simulink model "motor_control_SVPWM"  (R2023a)
settings: Solver=FixedStepAuto  StartTime=0.0  StopTime=10  FixedStep=1e-5  RelTol=1e-3
undefined symbols (not defined in the file): DiscIntNeverNeededParam
libraries: spsIGBTDiodeLib x6, simulink x3, spsCurrentMeasurementLib x3, spsAsynchronousMachineSIUnitsLib x1, spsDCVoltageSourceLib x1, slpidlib x1, spsTriangleGeneratorLib x1, sps_lib x1
settings Model: Creator=Vuong Thanh Tung  LastModifiedBy=Vuong Thanh Tung

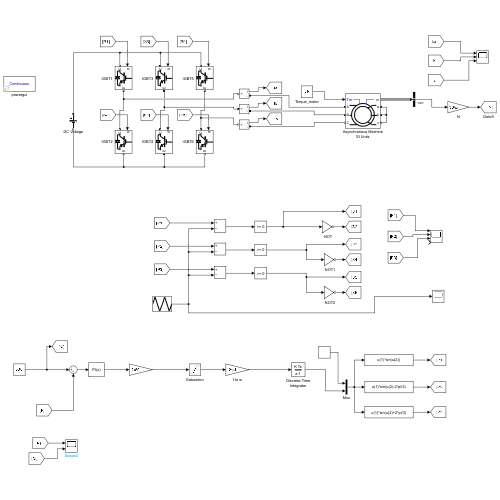
[thumbnail: Simulink's stored preview of the top-level diagram]
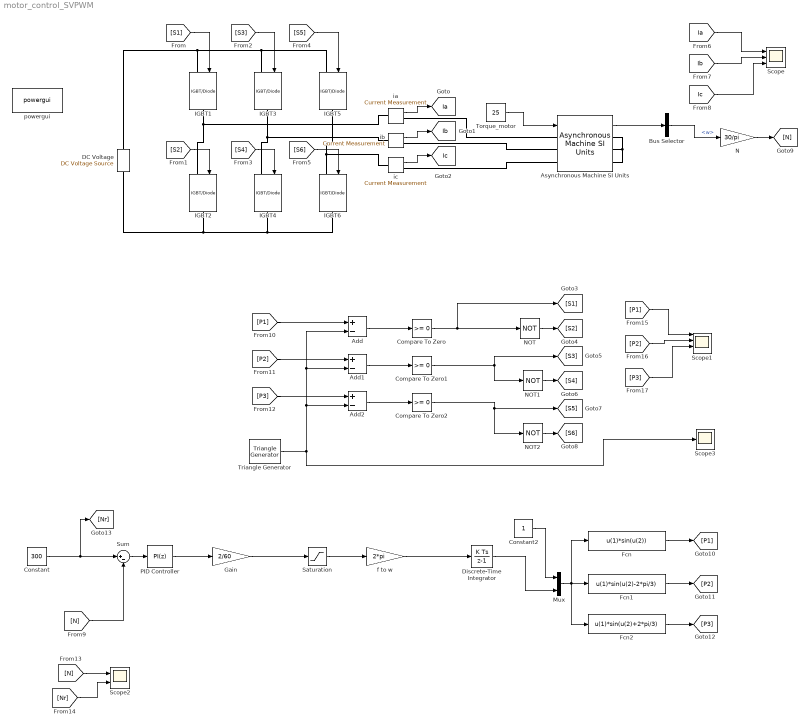
== system motor_control_SVPWM ==
  Add : Sum  Inputs=+-
  Add1 : Sum  Inputs=+-
  Add2 : Sum  Inputs=+-
  Asynchronous Machine SI Units : spsAsynchronousMachineSIUnitsLib/Asynchronous Machine SI Units  RotorType=Wound  PresetModel=No  MechanicalLoad=Torque Tm  ShowDetailedParameters=on  ReferenceFrame=Rotor  Units=SI  MeasurementBus=on  NominalParameters=[5e+03 400 50]  VoltageRatio=1  Stator=[0.5968 0.0003495]  Rotor=[0.6258 0.005473]  Cage1=[0.4155 0.002066]  Cage2=[0.4168 0.0003495]  Lm=0.0354  Mechanical=[0.05 0.005879 2]  PolePairs=2  InitialConditions=[0 0 0 0 0 0 0 0]  SimulateSaturation=off  Saturation=[14.03593122, 27.81365428, 53.79336849, 72.68890987, 97.98006896, 148.6815601, 215.7428561, 302.9841135, 428.7778367 ; 230, 322, 414, 460, 506, 552, 598, 644, 690]  LoadFlowParameters=1492000  TsPowergui=0  TsBlock=-1  IterativeModel=Trapezoidal non iterative  IterativeDiscreteModel=Trapezoidal non iterative  Pmec=55000
  Bus Selector : BusSelector  OutputSignals=w
  Compare To Zero : simulink/Logic and Bit Operations/Compare To Zero  relop=>=  OutDataTypeStr=boolean
  Compare To Zero1 : simulink/Logic and Bit Operations/Compare To Zero  relop=>=  OutDataTypeStr=boolean
  Compare To Zero2 : simulink/Logic and Bit Operations/Compare To Zero  relop=>=  OutDataTypeStr=boolean
  Constant : Constant  Value=300
  Constant2 : Constant
  DC Voltage : spsDCVoltageSourceLib/DC Voltage Source  Amplitude=380  Measurements=Voltage
  Discrete-Time Integrator : DiscreteIntegrator  SampleTime=-1  ICPrevOutput=DiscIntNeverNeededParam  ICPrevScaledInput=DiscIntNeverNeededParam
  Fcn : Fcn  Expr=u(1)*sin(u(2))
  Fcn1 : Fcn  Expr=u(1)*sin(u(2)-2*pi/3)
  Fcn2 : Fcn  Expr=u(1)*sin(u(2)+2*pi/3)
  Gain : Gain  Gain=2/60
  IGBT{1..6} (6 alike) : spsIGBTDiodeLib/IGBT//Diode  Ron=1e-3  Rs=1e5  Cs=inf  Measurements=off
  Mux : Mux  Inputs=2
  N : Gain  Gain=30/pi
  NOT : Logic  Operator=NOT  IconShape=distinctive  AllPortsSameDT=off  OutDataTypeStr=boolean
  NOT1 : Logic  Operator=NOT  IconShape=distinctive  AllPortsSameDT=off  OutDataTypeStr=boolean
  NOT2 : Logic  Operator=NOT  IconShape=distinctive  AllPortsSameDT=off  OutDataTypeStr=boolean
  PID Controller : slpidlib/PID Controller  Controller=PI  Form=Parallel  TimeDomain=Discrete-time  UseExternalTs=off  SampleTime=-1  IntegratorMethod=Forward Euler  FilterMethod=Forward Euler  ControllerParametersSource=internal  P=0.7  I=0.4  UseKiTs=off  D=0  N=100  UseFilter=on  TunerSelectOption=Transfer Function Based (PID Tuner App)  InitialConditionSource=internal  InitialConditionForIntegrator=0  InitialConditionForFilter=0  DifferentiatorICPrevScaledInput=0  ExternalReset=none  TrackingMode=off  Kt=1  LimitOutput=off  SatLimitsSource=internal  UpperSaturationLimit=inf  LowerSaturationLimit=-inf  LinearizeAsGain=on  AntiWindupMode=none  Kb=1  LimitIntegrator=off  UpperIntegratorSaturationLimit=inf  LowerIntegratorSaturationLimit=-inf  POutMin=[]  POutMax=[]  IOutMin=[]  IOutMax=[]  DOutMin=[]  DOutMax=[]  NOutMin=[]  NOutMax=[]  SumOutMin=[]  SumOutMax=[]  SaturationOutMin=[]  SaturationOutMax=[]  PParamMin=[]  PParamMax=[]  IParamMin=[]  IParamMax=[]  DParamMin=[]  DParamMax=[]  NParamMin=[]  NParamMax=[]  KbParamMin=[]  KbParamMax=[]  KtParamMin=[]  KtParamMax=[]  KbOutMin=[]  KbOutMax=[]  KtOutMin=[]  KtOutMax=[]  IntegratorOutMin=[]  IntegratorOutMax=[]  FilterOutMin=[]  FilterOutMax=[]  SumI1OutMin=[]  SumI1OutMax=[]  SumI2OutMin=[]  SumI2OutMax=[]  SumI3OutMin=[]  SumI3OutMax=[]  SumI4OutMin=[]  SumI4OutMax=[]  SumDOutMin=[]  SumDOutMax=[]  DifferentiatorOutMin=[]  DifferentiatorOutMax=[]  FilterDiffOutCoefMin=[]  FilterDiffOutCoefMax=[]  ReciprocalOutMin=[]  ReciprocalOutMax=[]  SumDenOutMin=[]  SumDenOutMax=[]  SumNumOutMin=[]  SumNumOutMax=[]  DivideOutMin=[]  DivideOutMax=[]  UdiffTsProdOutMin=[]  UdiffTsProdOutMax=[]  NTsProdOutMin=[]  NTsProdOutMax=[]  UintegralTsProdOutMin=[]  UintegralTsProdOutMax=[]  UngainTsProdOutMin=[]  UngainTsProdOutMax=[]  ClampingZeroOutDataTypeStr=Inherit: Inherit via back propagation  ClampingZeroOutMin=[]  ClampingZeroOutMax=[]  FilterDenConstantOutDataTypeStr=Inherit: Inherit via back propagation  FilterDenConstantOutMin=[]  FilterDenConstantOutMax=[]  PCopyOutDataTypeStr=Inherit: Inherit via back propagation  PCopyOutMin=[]  PCopyOutMax=[]  NCopyOutDataTypeStr=Inherit: Inherit via back propagation  NCopyOutMin=[]  NCopyOutMax=[]  IntegratorContinuousStateAttributes=''  IntegratorStateMustResolveToSignalObject=off  IntegratorRTWStateStorageClass=Auto  FilterContinuousStateAttributes=''  FilterStateMustResolveToSignalObject=off  FilterRTWStateStorageClass=Auto  ParallelPVariant=InternalParameters  IdealPVariant=Disabled  IVariant=InternalParameters  DVariant=Disabled  IntegratorVariant=Discrete  SatVariant=Disabled  AWVariant=Passthrough  PCopyVariant=Disabled  TRVariant=Disabled  FdbkBlocksVariant=Forward  IdealPFdbkVariant=Disabled  SatFdbkVariant=Disabled  DerivativeFilterVariant=Disabled  NVariant=Disabled  NCopyVariant=Disabled_SignalSpec  FilterICVariant=Disabled  IntegratorICVariant=InternalICs  ExternalResetVariant=Disabled  TRSumVariant=Passthrough  SumFdbkVariant=Disabled  SumVariant=Sum_PI  TsampFilterVariant=InternalTs  TsampNgainVariant=Passthrough  TsampIntegralVariant=Disabled_SignalSpec  ExternalSaturationOutDataTypeStr=Inherit: Same as second input
  Saturation : Saturate  UpperLimit=100  LowerLimit=0
  Scope : Scope  NumInputPorts=3
  Scope1 : Scope  NumInputPorts=4
  Scope2 : Scope  NumInputPorts=2
  Scope3 : Scope
  Sum : Sum  Inputs=|+-
  Torque_motor : Constant  Value=25
  Triangle Generator : spsTriangleGeneratorLib/Triangle Generator  Freq=200  Phase=90  Ts=0
  f to w : Gain  Gain=2*pi
  ia : spsCurrentMeasurementLib/Current Measurement  PhasorSimulation=off  OutputType=Complex  PSBequivalent=0
  ib : spsCurrentMeasurementLib/Current Measurement  PhasorSimulation=off  OutputType=Complex  PSBequivalent=0
  ic : spsCurrentMeasurementLib/Current Measurement  PhasorSimulation=off  OutputType=Complex  PSBequivalent=0
  powergui : sps_lib/powergui  Priority=1  SimulationMode=Continuous  SampleTime=50e-6  frequency=60  Iterations=50  frequencyindice=50  Pbase=100e6  ErrMax=1e-4  UnitsV=kV  UnitsW=MW  buscounter=0  FunctionMessages=off  echomessages=off  EnableUseOfTLC=off  CurrentSourceSwitches=off  DisableSnubberDevices=off  DisableRonSwitches=off  DisableVfSwitches=off  DisplayEquations=off  AutomaticDiscreteSolvers=off  SolverType=Tustin/Backward Euler (TBE)  Interpol=off  ExternalGateDelay=off  methode=off  Ts=100  x0status=blocks  SPID=on  SwTol=0  HookPort=off  NonlinearTolerance=1e-4  nMaxIteration=100  ContinueOnMaxIteration=off  RestoreLinks=warning  ResistiveCurrentMeasurement=off  Frange=[0:2:500]  Ylog=off  Xlog=on  ShowGrid=off  save=off  variable=ZData  structure=0  ZoomFFT=off  StartTime=0.0  cycles=1  DisplayStyle=1  fundamental=60  FreqAxis=off  MaxFrequency=1000  frequencyindicesteady=1  RmsSteady=1  display=off
  tag scope: Ia=global, Ib=global, Ic=global
  wires:
  ic/1 -> [Ic]
  ib/1 -> [Ib]
  ia/1 -> [Ia]
  Torque_motor/1 -> Asynchronous Machine SI Units/1
  [S1] -> IGBT1/1
  [S2] -> IGBT2/1
  [S3] -> IGBT3/1
  [S4] -> IGBT4/1
  [S5] -> IGBT5/1
  [S6] -> IGBT6/1
  NOT/1 -> [S2]
  NOT1/1 -> [S4]
  NOT2/1 -> [S6]
  Asynchronous Machine SI Units/1 -> Bus Selector/1
  Bus Selector/1 -> N/1  "<w>"
  N/1 -> [N]
  Add/1 -> Compare To Zero/1
  Compare To Zero/1 -> NOT/1, [S1]
  Add1/1 -> Compare To Zero1/1
  Add2/1 -> Compare To Zero2/1
  Compare To Zero1/1 -> NOT1/1, [S3]
  Compare To Zero2/1 -> NOT2/1, [S5]
  [Ia] -> Scope/1
  [Ib] -> Scope/2
  [Ic] -> Scope/3
  Triangle Generator/1 -> Add2/2, Add1/2, Add/2, Scope3/1
  [P1] -> Add/1
  [P3] -> Add2/1
  [P2] -> Add1/1
  Constant/1 -> [Nr], Sum/1
  Sum/1 -> PID Controller/1
  [N] -> Sum/2
  PID Controller/1 -> Gain/1
  Saturation/1 -> f to w/1
  f to w/1 -> Discrete-Time Integrator/1
  Discrete-Time Integrator/1 -> Mux/2
  Mux/1 -> Fcn2/1, Fcn/1, Fcn1/1
  Fcn/1 -> [P1]
  Fcn1/1 -> [P2]
  Fcn2/1 -> [P3]
  [N] -> Scope2/1
  [Nr] -> Scope2/2
  [P1] -> Scope1/1
  [P2] -> Scope1/2
  [P3] -> Scope1/3
  Constant2/1 -> Mux/1
  Gain/1 -> Saturation/1
  connections:
  IGBT1/RConn1 -- ia/LConn1 -- IGBT2/LConn1
  IGBT3/RConn1 -- ib/LConn1 -- IGBT4/LConn1
  IGBT5/RConn1 -- ic/LConn1 -- IGBT6/LConn1
  IGBT1/LConn1 -- DC Voltage/RConn1 -- IGBT3/LConn1 -- IGBT5/LConn1
  IGBT2/RConn1 -- DC Voltage/LConn1 -- IGBT4/RConn1 -- IGBT6/RConn1
  ia/RConn1 -- Asynchronous Machine SI Units/LConn1
  ib/RConn1 -- Asynchronous Machine SI Units/LConn2
  ic/RConn1 -- Asynchronous Machine SI Units/LConn3
  Asynchronous Machine SI Units/RConn3 -- Asynchronous Machine SI Units/RConn1 -- Asynchronous Machine SI Units/RConn2
